simulink model "PX4ExtMsgSender"  (R2020b)
settings: Solver=ode4  StartTime=0.0  StopTime=inf  FixedStep=0.005  RelTol=1e-3
PreLoadFcn:
  | filepath  = fileparts(get_param(bdroot, 'FileName'))
  | cd(filepath);
undefined symbols (not defined in the file or in its folder): Busy, Earth, Wait, WGS84
libraries: etargetslib x6, slrealtimeiplib x3, dspnetwork x2, aerolibanimutils x1, aerolibtransform2 x1
settings Model: SimulationMode=accelerator  Creator=dream  LastModifiedBy=dzl20201126
settings DataIOCC: ReturnWorkspaceOutputs=off
settings DebuggingCC: ArithmeticOperatorsInVariantConditions=warning
settings SFSimCC: SimUseLocalCustomCode=off  CustomCodeUndefinedFunction=UseInterfaceOnly
settings RTWCC: RTWUseLocalCustomCode=off

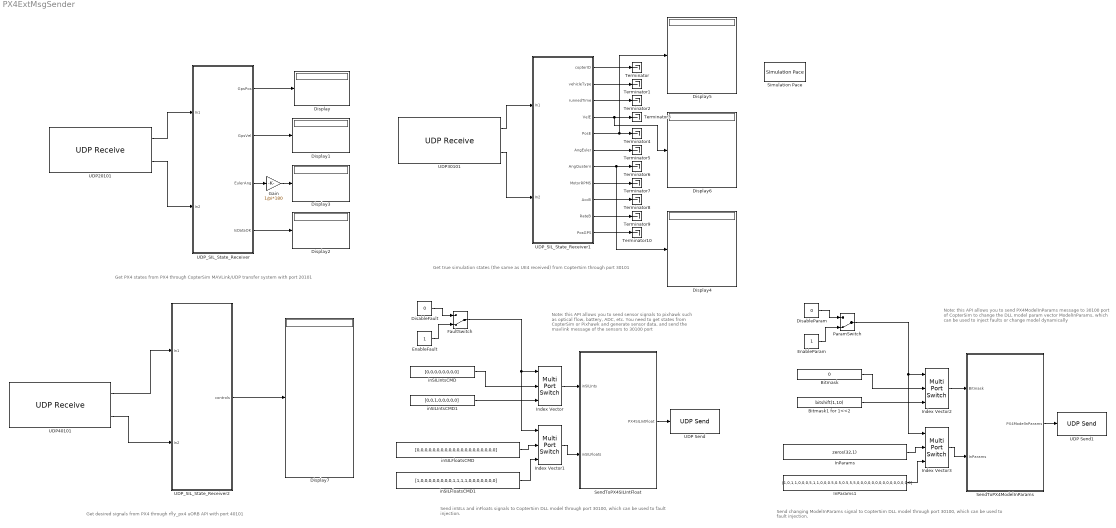
== system PX4ExtMsgSender ==
  note: Get PX4 states from PX4 through CopterSim MAVLink/UDP transfer system with port 20101
  note: Get true simulation states (the same as UE4 received) from CopterSim through port 30101
  note: Get desired signals from PX4 through rfly_px4 uORB API with port 40101
  note: Send inSILs and inFloats signals to CopterSim DLL model through port 30100, which can be used to fault injection.
  note: Note: this API allows you to send sensor signals to pixhawk such as optical flow, battery, ADC, etc. You need to get states from CopterSim or Pixhawk and generate sensor data, and send the mavlink message of the sensors to 30100 port
  note: Note: this API allows you to send PX4ModelInParams message to 30100 port of CopterSim to change the DLL model param vector ModelInParams, which can be used to inject faults or change model dynamically
  note: Send changing ModelInParams signal to CopterSim DLL model through port 30100, which can be used to fault injection.
  Bitmask : Constant  Value=0  OutDataTypeStr=int32
  Bitmask1 for 1<<2 : Constant  Value=bitshift(1,10)  OutDataTypeStr=int32
  DisableFault : Constant  Value=0
  DisableParam : Constant  Value=0
  Display{,1..7} (8 alike) : Display
  EnableFault : Constant
  EnableParam : Constant
  FaultSwitch : ManualSwitch  CurrentSetting=0
  Gain : Gain  Gain=1/pi*180
  InParams : Constant  Value=zeros(32,1)  OutDataTypeStr=single
  InParams1 : Constant  Value=[1,0,1,1,0,0,0,5,1,1,0,0,0.5,0.5,0.5,5,5,0,0,0,0,0,0,0,0,0,0,0,0,0,0,0]  OutDataTypeStr=single
  Index Vector{,1..3} (4 alike) : MultiPortSwitch  DataPortOrder=Zero-based contiguous  Inputs=2  zeroidx=on
  ParamSwitch : ManualSwitch  CurrentSetting=0
  SendToPX4ModelInParams : Subsystem
  SendToPX4SILIntFloat : Subsystem
  Simulation Pace : aerolibanimutils/Simulation Pace  SimulationPace=1  SleepMode=Busy-Wait  OutputPaceError=off  SampleTime=-1
  Terminator{,1..10} (11 alike) : Terminator
  UDP Send : dspnetwork/UDP Send  remoteURL='127.0.0.1'  remotePort=30100  localURL='0.0.0.0'  localPortSource=Automatically determine  localPort=-1  sendBufferSize=8192  sampletime=-1  blockPlatform=[]  separateLengthPort=0
  UDP Send1 : dspnetwork/UDP Send  remoteURL='127.0.0.1'  remotePort=30100  localURL='0.0.0.0'  localPortSource=Automatically determine  localPort=-1  sendBufferSize=8192  sampletime=-1  blockPlatform=[]  separateLengthPort=0
  UDP20101 : slrealtimeiplib/UDP Receive  useHostTargetConn=on  ipAddress=10.10.10.15  localPort=20101  rcvWidth=125  rcvFmAny=on  fmAddress=0.0.0.0  rcvMulticast=off  multicastAddress={}  sampleTime=-1
      settings: SourceProductBaseCode=XP
  UDP30101 : slrealtimeiplib/UDP Receive  useHostTargetConn=on  ipAddress=10.10.10.15  localPort=30101  rcvWidth=250  rcvFmAny=on  fmAddress=0.0.0.0  rcvMulticast=off  multicastAddress={}  sampleTime=-1
      settings: SourceProductBaseCode=XP
  UDP40101 : slrealtimeiplib/UDP Receive  useHostTargetConn=on  ipAddress=10.10.10.15  localPort=40101  rcvWidth=120  rcvFmAny=on  fmAddress=0.0.0.0  rcvMulticast=off  multicastAddress={}  sampleTime=-1
      settings: SourceProductBaseCode=XP
  UDP_SIL_State_Receiver : Subsystem
  UDP_SIL_State_Receiver1 : Subsystem
  UDP_SIL_State_Receiver2 : Subsystem
  inSILFloatsCMD : Constant  Value=[0,0,0,0,0,0,0,0,0,0,0,0,0,0,0,0,0,0,0,0]  OutDataTypeStr=single
  inSILFloatsCMD1 : Constant  Value=[1,0,0,0,0,0,0,0,0,1,1,1,1,0,0,0,0,0,0,0]  OutDataTypeStr=single
  inSILIntsCMD : Constant  Value=[0,0,0,0,0,0,0,0]  OutDataTypeStr=int32
  inSILIntsCMD1 : Constant  Value=[0,0,1,0,0,0,0,0]  OutDataTypeStr=int32
  wires:
  UDP20101/1 -> UDP_SIL_State_Receiver/1(In1)
  UDP20101/2 -> UDP_SIL_State_Receiver/2(In2)
  UDP_SIL_State_Receiver/1(GpsPos) -> Display/1
  UDP_SIL_State_Receiver/2(GpsVel) -> Display1/1
  UDP_SIL_State_Receiver/3(EulerAng) -> Gain/1
  Gain/1 -> Display3/1
  UDP_SIL_State_Receiver/4(IsDataOK) -> Display2/1
  UDP_SIL_State_Receiver1/8(MotorRPMS) -> Terminator7/1
  UDP_SIL_State_Receiver1/2(vehicleType) -> Terminator1/1
  UDP_SIL_State_Receiver1/9(AccB) -> Terminator8/1
  UDP_SIL_State_Receiver1/11(PosGPS) -> Terminator10/1
  UDP30101/2 -> UDP_SIL_State_Receiver1/2(In2)
  UDP_SIL_State_Receiver1/5(PosE) -> Display5/1, Terminator4/1
  UDP_SIL_State_Receiver1/6(AngEuler) -> Terminator5/1
  UDP_SIL_State_Receiver1/7(AngQuatern) -> Display4/1, Terminator6/1
  UDP_SIL_State_Receiver1/4(VelE) -> Display6/1, Terminator3/1
  SendToPX4SILIntFloat/1(PX4SILIntFloat) -> UDP Send/1
  UDP_SIL_State_Receiver1/3(runnedTime) -> Terminator2/1
  UDP_SIL_State_Receiver1/1(copterID) -> Terminator/1
  Index Vector1/1 -> SendToPX4SILIntFloat/2(inSILFloats)
  UDP30101/1 -> UDP_SIL_State_Receiver1/1(In1)
  DisableFault/1 -> FaultSwitch/1
  inSILFloatsCMD/1 -> Index Vector1/2
  inSILFloatsCMD1/1 -> Index Vector1/3
  Index Vector/1 -> SendToPX4SILIntFloat/1(inSILInts)
  inSILIntsCMD/1 -> Index Vector/2
  UDP_SIL_State_Receiver1/10(RateB) -> Terminator9/1
  EnableFault/1 -> FaultSwitch/2
  FaultSwitch/1 -> Index Vector1/1, Index Vector/1
  inSILIntsCMD1/1 -> Index Vector/3
  UDP40101/1 -> UDP_SIL_State_Receiver2/1(In1)
  UDP40101/2 -> UDP_SIL_State_Receiver2/2(In2)
  UDP_SIL_State_Receiver2/1(controls) -> Display7/1
  Index Vector2/1 -> SendToPX4ModelInParams/1(Bitmask)
  Bitmask1 for 1<<2/1 -> Index Vector2/3
  InParams/1 -> Index Vector3/2
  EnableParam/1 -> ParamSwitch/2
  InParams1/1 -> Index Vector3/3
  Bitmask/1 -> Index Vector2/2
  DisableParam/1 -> ParamSwitch/1
  ParamSwitch/1 -> Index Vector3/1, Index Vector2/1
  SendToPX4ModelInParams/1(PX4ModelInParams) -> UDP Send1/1
  Index Vector3/1 -> SendToPX4ModelInParams/2(InParams)

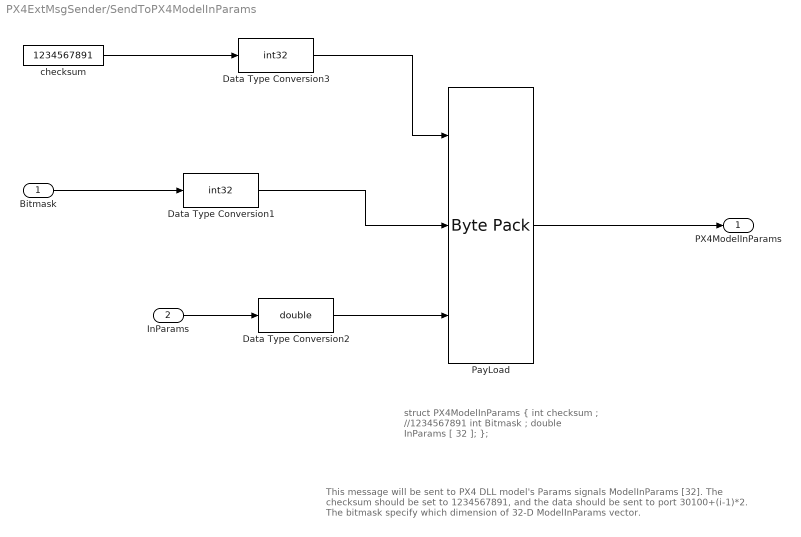
== system PX4ExtMsgSender/SendToPX4ModelInParams ==
  note: struct PX4ModelInParams {
      | int checksum ; //1234567891
      | int Bitmask ;
      | double InParams [ 32 ];
      | };
  note: This message will be sent to PX4 DLL model's Params signals ModelInParams [32].
      | The checksum should be set to 1234567891, and the data should be sent to port 30100+(i-1)*2.
      | The bitmask specify which dimension of 32-D ModelInParams vector.
  Bitmask : Inport  OutDataTypeStr=int32  PortDimensions=1
  InParams : Inport  Port=2  OutDataTypeStr=single  PortDimensions=32
  Data Type Conversion1 : DataTypeConversion  OutDataTypeStr=int32
  Data Type Conversion2 : DataTypeConversion  OutDataTypeStr=double
  Data Type Conversion3 : DataTypeConversion  OutDataTypeStr=int32
  PayLoad : etargetslib/Byte Pack  datatypes={'int32','int32','double'}  byteAlign=4
  checksum : Constant  Value=1234567891  OutDataTypeStr=Inherit: Inherit via back propagation
  PX4ModelInParams : Outport  OutDataTypeStr=uint8  VectorParamsAs1DForOutWhenUnconnected=off
  wires:
  InParams/1 -> Data Type Conversion2/1
  Bitmask/1 -> Data Type Conversion1/1
  PayLoad/1 -> PX4ModelInParams/1
  Data Type Conversion1/1 -> PayLoad/2
  Data Type Conversion2/1 -> PayLoad/3
  checksum/1 -> Data Type Conversion3/1
  Data Type Conversion3/1 -> PayLoad/1

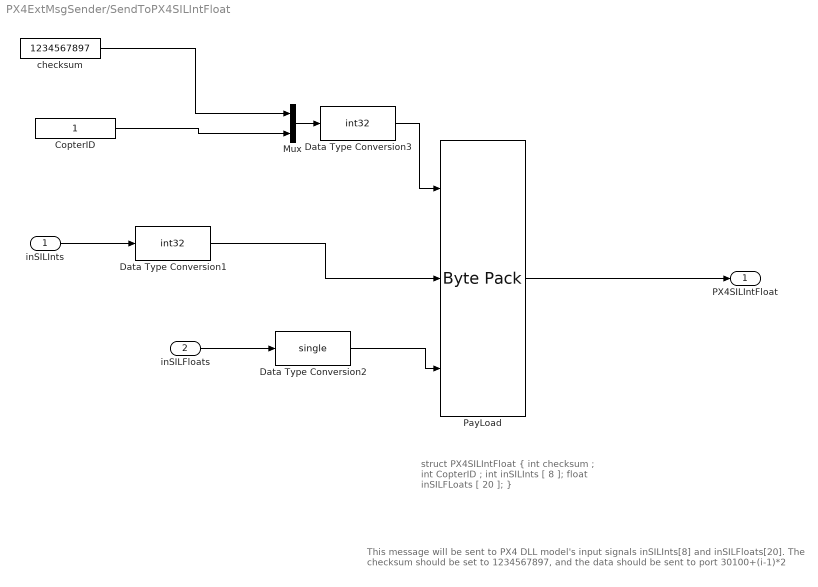
== system PX4ExtMsgSender/SendToPX4SILIntFloat ==
  note: struct PX4SILIntFloat {
      | int checksum ;
      | int CopterID ;
      | int inSILInts [ 8 ];
      | float inSILFLoats [ 20 ];
      | }
  note: This message will be sent to PX4 DLL model's input signals inSILInts[8] and inSILFloats[20].
      | The checksum should be set to 1234567897, and the data should be sent to port 30100+(i-1)*2
  inSILInts : Inport  OutDataTypeStr=int32  PortDimensions=8
  inSILFloats : Inport  Port=2  OutDataTypeStr=single  PortDimensions=20
  CopterID : Constant  OutDataTypeStr=Inherit: Inherit via back propagation
  Data Type Conversion1 : DataTypeConversion  OutDataTypeStr=int32
  Data Type Conversion2 : DataTypeConversion  OutDataTypeStr=single
  Data Type Conversion3 : DataTypeConversion  OutDataTypeStr=int32
  Mux : Mux  Inputs=2
  PayLoad : etargetslib/Byte Pack  datatypes={'int32','int32','single'}  byteAlign=8
  checksum : Constant  Value=1234567897  OutDataTypeStr=Inherit: Inherit via back propagation
  PX4SILIntFloat : Outport  OutDataTypeStr=uint8  PortDimensions=120  VectorParamsAs1DForOutWhenUnconnected=off
  wires:
  inSILFloats/1 -> Data Type Conversion2/1
  inSILInts/1 -> Data Type Conversion1/1
  PayLoad/1 -> PX4SILIntFloat/1
  Data Type Conversion1/1 -> PayLoad/2
  Data Type Conversion2/1 -> PayLoad/3
  checksum/1 -> Mux/1
  Mux/1 -> Data Type Conversion3/1
  Data Type Conversion3/1 -> PayLoad/1
  CopterID/1 -> Mux/2

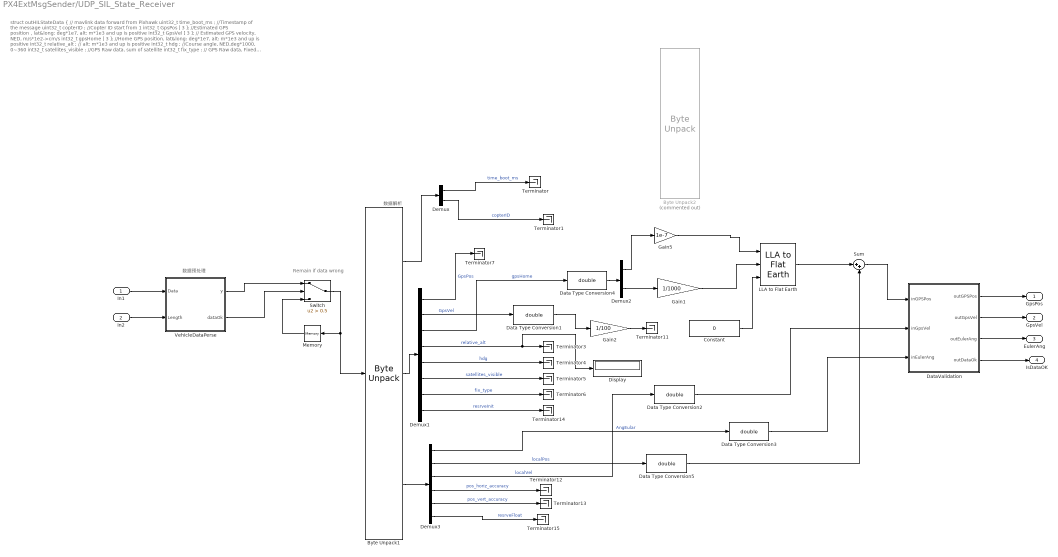
== system PX4ExtMsgSender/UDP_SIL_State_Receiver ==
  note: 数据解析
  note: 数据预处理
  note: Remain if data wrong
  note: struct outHILStateData { // mavlink data forward from Pixhawk
      | uint32_t time_boot_ms ; //Timestamp of the message
      | uint32_t copterID ; //Copter ID start from 1
      | int32_t GpsPos [ 3 ]; //Estimated GPS position，lat&long: deg*1e7, alt: m*1e3 and up is positive
      | int32_t GpsVel [ 3 ]; // Estimated GPS velocity, NED, m/s*1e2->cm/s
      | int32_t gpsHome [ 3 ]; //Home GPS position, lat&long: deg*1e7, alt: m*1e3 and up is positive
      | int32_t relative_alt ; // alt: m*1e3 and up is positive
      | int32_t hdg ; //Course angle, NED,deg*1000, 0~360
      | int32_t satellites_visible ; //GPS Raw data, sum of satellite
      | int32_t fix_type ; // GPS Raw data, Fixed type, 3 for fixed (good precision)
      | int32_t resrveInit ; //Int, reserve for the future use
      | float AngEular [ 3 ]; //Estimated Euler angle, unit: rad/s
      | float localPos [ 3 ]; //Estimated locoal position, NED, unit: m
      | float localVel [ 3 ]; // Estimated locoal velocity, NED, unit: m/s
      | float pos_horiz_accuracy ; // GPS horizontal accuracy, unit: m
      | float pos_vert_accuracy ; // GPS vertical accuracy, unit: m
      | float resrveFloat ; //float, reserve for the future use
      | }
  In1 : Inport
  In2 : Inport  Port=2
  Byte Unpack1 : etargetslib/Byte Unpack  dimensions={2,14,12}  datatypes={'uint32','int32','single'}  byteAlign=8
  Byte Unpack2 : etargetslib/Byte Unpack  Commented=on  dimensions={1,1,1,3,3,3,4,8,3,3,3}  datatypes={'int32','int32','double','single','single','single','single','single','single','single','double'}  byteAlign=1
  Constant : Constant  Value=0
  Data Type Conversion{1..5} (5 alike) : DataTypeConversion  OutDataTypeStr=double
  DataValidation : MATLAB Function  TreatAsAtomicUnit=on
  Demux : Demux  Outputs=2
  Demux1 : Demux  Outputs=[3,3,3,1,1,1,1,1]
  Demux2 : Demux  Outputs=[2,1]
  Demux3 : Demux  Outputs=[3,3,3,1,1,1]
  Display : Display
  Gain1 : Gain  Gain=1/1000
  Gain2 : Gain  Gain=1/100
  Gain5 : Gain  Gain=1e-7
  LLA to Flat Earth : aerolibtransform2/LLA to Flat Earth  units=Metric (MKS)  ptype=Earth (WGS84)  F=1/298.257223563  R=6378137  refPosPort=off  LL0=[40.1540302 116.259368300000]  psi=0
      settings: SourceProductBaseCode=AE
  Memory : Memory  InitialCondition=uint8(zeros(112,1))
  Sum : Sum  Inputs=|++
  Switch : Switch  Criteria=u2 > Threshold  Threshold=0.5
  Terminator{,1,3..7,11..15} (12 alike) : Terminator
  VehicleDataPerse : MATLAB Function  TreatAsAtomicUnit=on
  GpsPos : Outport  VectorParamsAs1DForOutWhenUnconnected=off
  GpsVel : Outport  Port=2  VectorParamsAs1DForOutWhenUnconnected=off
  EulerAng : Outport  Port=3  VectorParamsAs1DForOutWhenUnconnected=off
  IsDataOK : Outport  Port=4  VectorParamsAs1DForOutWhenUnconnected=off
  wires:
  VehicleDataPerse/2(dataOk) -> Switch/2
  In2/1 -> VehicleDataPerse/2(Length)
  In1/1 -> VehicleDataPerse/1(Data)
  VehicleDataPerse/1(y) -> Switch/1
  Switch/1 -> Memory/1, Byte Unpack1/1
  Memory/1 -> Switch/3
  Byte Unpack1/1 -> Demux/1
  Demux/1 -> Terminator/1  "time_boot_ms"
  Demux/2 -> Terminator1/1  "copterID"
  Byte Unpack1/2 -> Demux1/1
  Demux1/2 -> Data Type Conversion1/1  "GpsVel"
  Demux2/1 -> Gain5/1
  Demux2/2 -> Gain1/1
  Gain1/1 -> LLA to Flat Earth/2
  Demux1/1 -> Terminator7/1  "GpsPos"
  LLA to Flat Earth/1 -> Sum/1
  Data Type Conversion1/1 -> Gain2/1
  Data Type Conversion3/1 -> DataValidation/3(inEulerAng)
  Gain5/1 -> LLA to Flat Earth/1
  Data Type Conversion4/1 -> Demux2/1
  Byte Unpack1/3 -> Demux3/1
  Demux1/3 -> Data Type Conversion4/1  "gpsHome"
  Demux1/4 -> Display/1, Terminator3/1  "relative_alt"
  Demux1/5 -> Terminator4/1  "hdg"
  Demux1/6 -> Terminator5/1  "satellites_visible"
  Demux1/7 -> Terminator6/1  "fix_type"
  Demux3/1 -> Data Type Conversion3/1  "AngEular"
  Demux3/2 -> Data Type Conversion5/1  "localPos"
  Demux3/3 -> Data Type Conversion2/1  "localVel"
  Demux3/4 -> Terminator12/1  "pos_horiz_accuracy"
  Demux3/5 -> Terminator13/1  "pos_vert_accuracy"
  Demux1/8 -> Terminator14/1  "resrveInit"
  Demux3/6 -> Terminator15/1  "resrveFloat"
  Constant/1 -> LLA to Flat Earth/3
  DataValidation/1(outGPSPos) -> GpsPos/1
  DataValidation/2(outGpsVel) -> GpsVel/1
  DataValidation/3(outEulerAng) -> EulerAng/1
  DataValidation/4(outDataOk) -> IsDataOK/1
  Data Type Conversion2/1 -> DataValidation/2(inGpsVel)
  Gain2/1 -> Terminator11/1
  Data Type Conversion5/1 -> Sum/2
  Sum/1 -> DataValidation/1(inGPSPos)

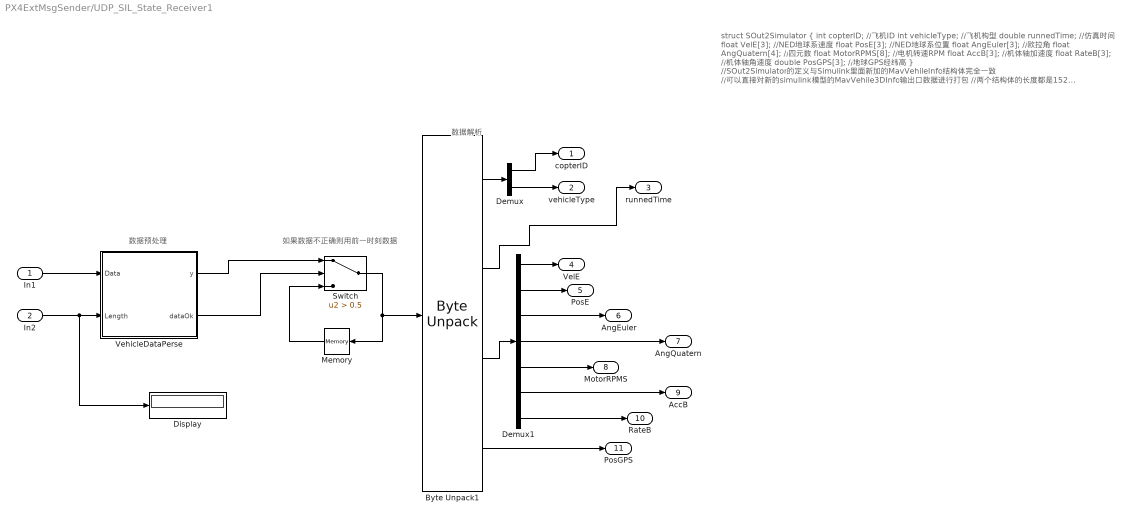
== system PX4ExtMsgSender/UDP_SIL_State_Receiver1 ==
  note: 数据解析
  note: 数据预处理
  note: 如果数据不正确则用前一时刻数据
  note: struct SOut2Simulator
      | {
      | int copterID; //飞机ID
      | int vehicleType; //飞机构型
      | double runnedTime; //仿真时间
      | float VelE[3]; //NED地球系速度
      | float PosE[3]; //NED地球系位置
      | float AngEuler[3]; //欧拉角
      | float AngQuatern[4]; //四元数
      | float MotorRPMS[8]; //电机转速RPM
      | float AccB[3]; //机体轴加速度
      | float RateB[3]; //机体轴角速度
      | double PosGPS[3]; //地球GPS经纬高
      | }
      |
      | //SOut2Simulator的定义与Simulink里面新加的MavVehileInfo结构体完全一致
      | //可以直接对新的simulink模型的MavVehile3DInfo输出口数据进行打包
      | //两个结构体的长度都是152
      | sizeof(SOut2Simulator) = sizeof(MavVehileInfo) = 152
      |
      | 打包封装的结构体为
      | typedef struct _netDataShort
      | {
      | TargetType tg; //这里目前随便填，写1即可 uint32
      | int len; //这个长度为传输结构体长度，目前是152
      | char payload[192]; //这里面前152位存放了SOut2Simulator结构体数据，后面的40位保留
      | }netDataShort;
      |
      | //UDP包的总长度为200
      | sizeof(netDataShort) = 200
      |
      | //发送的UDP端口号为：20010
  In1 : Inport
  In2 : Inport  Port=2
  Byte Unpack1 : etargetslib/Byte Unpack  dimensions={2,1,27,3}  datatypes={'int32','double','single','double'}  byteAlign=8
  Demux : Demux  Outputs=2
  Demux1 : Demux  Outputs=[3,3,3,4,8,3,3]
  Display : Display
  Memory : Memory  InitialCondition=uint8(zeros(152,1))
  Switch : Switch  Criteria=u2 > Threshold  Threshold=0.5
  VehicleDataPerse : MATLAB Function  TreatAsAtomicUnit=on
  copterID : Outport  VectorParamsAs1DForOutWhenUnconnected=off
  vehicleType : Outport  Port=2  VectorParamsAs1DForOutWhenUnconnected=off
  runnedTime : Outport  Port=3  VectorParamsAs1DForOutWhenUnconnected=off
  VelE : Outport  Port=4  VectorParamsAs1DForOutWhenUnconnected=off
  PosE : Outport  Port=5  VectorParamsAs1DForOutWhenUnconnected=off
  AngEuler : Outport  Port=6  VectorParamsAs1DForOutWhenUnconnected=off
  AngQuatern : Outport  Port=7  VectorParamsAs1DForOutWhenUnconnected=off
  MotorRPMS : Outport  Port=8  VectorParamsAs1DForOutWhenUnconnected=off
  AccB : Outport  Port=9  VectorParamsAs1DForOutWhenUnconnected=off
  RateB : Outport  Port=10  VectorParamsAs1DForOutWhenUnconnected=off
  PosGPS : Outport  Port=11  VectorParamsAs1DForOutWhenUnconnected=off
  wires:
  VehicleDataPerse/2(dataOk) -> Switch/2
  In2/1 -> Display/1, VehicleDataPerse/2(Length)
  In1/1 -> VehicleDataPerse/1(Data)
  VehicleDataPerse/1(y) -> Switch/1
  Switch/1 -> Memory/1, Byte Unpack1/1
  Memory/1 -> Switch/3
  Byte Unpack1/1 -> Demux/1
  Demux/1 -> copterID/1
  Demux/2 -> vehicleType/1
  Byte Unpack1/2 -> runnedTime/1
  Byte Unpack1/3 -> Demux1/1
  Demux1/1 -> VelE/1
  Demux1/2 -> PosE/1
  Demux1/3 -> AngEuler/1
  Demux1/4 -> AngQuatern/1
  Demux1/5 -> MotorRPMS/1
  Demux1/6 -> AccB/1
  Demux1/7 -> RateB/1
  Byte Unpack1/4 -> PosGPS/1

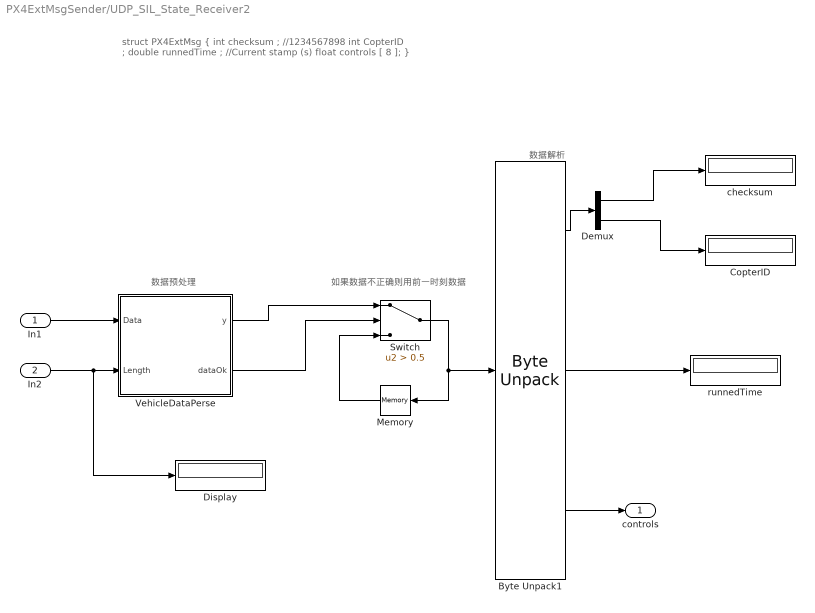
== system PX4ExtMsgSender/UDP_SIL_State_Receiver2 ==
  note: struct PX4ExtMsg {
      | int checksum ; //1234567898
      | int CopterID ;
      | double runnedTime ; //Current stamp (s)
      | float controls [ 8 ];
      | }
  note: 数据解析
  note: 数据预处理
  note: 如果数据不正确则用前一时刻数据
  In1 : Inport
  In2 : Inport  Port=2
  Byte Unpack1 : etargetslib/Byte Unpack  dimensions={2,1,8}  datatypes={'int32','double','single'}  byteAlign=8
  CopterID : Display
  Demux : Demux  Outputs=2
  Display : Display
  Memory : Memory  InitialCondition=uint8(zeros(48,1))
  Switch : Switch  Criteria=u2 > Threshold  Threshold=0.5
  VehicleDataPerse : MATLAB Function  TreatAsAtomicUnit=on
  checksum : Display
  runnedTime : Display
  controls : Outport  VectorParamsAs1DForOutWhenUnconnected=off
  wires:
  VehicleDataPerse/2(dataOk) -> Switch/2
  In2/1 -> Display/1, VehicleDataPerse/2(Length)
  In1/1 -> VehicleDataPerse/1(Data)
  VehicleDataPerse/1(y) -> Switch/1
  Switch/1 -> Memory/1, Byte Unpack1/1
  Memory/1 -> Switch/3
  Byte Unpack1/1 -> Demux/1
  Demux/1 -> checksum/1
  Demux/2 -> CopterID/1
  Byte Unpack1/2 -> runnedTime/1
  Byte Unpack1/3 -> controls/1

== matlab function PX4ExtMsgSender/UDP_SIL_State_Receiver1/VehicleDataPerse ==
  data: Data input; y output uint8 size=[152,1]; Length input; dataOk output
function [y,dataOk] = fcn(Data,Length)
y=uint8(zeros(152,1));
dataOk = 0;
if Length ~= 200
    return;
end
len = typecast(Data(5:8), 'int32');

if len ~= 152
   return; 
end

y = Data(9:160);
dataOk = 1;

== matlab function PX4ExtMsgSender/UDP_SIL_State_Receiver/DataValidation ==
  data: inGPSPos input; outGPSPos output; inGpsVel input; inEulerAng input; outGpsVel output; outEulerAng output; outDataOk output
function [outGPSPos,outGpsVel,outEulerAng,outDataOk] = fcn(inGPSPos,inGpsVel,inEulerAng)

outGPSPos = [0;0;0];
outGpsVel = [0;0;0];
outEulerAng = [0;0;0];
outDataOk = 0;

if(abs(inGPSPos(1))<10000)
    outGPSPos=inGPSPos;
    outGpsVel=inGpsVel;
    outEulerAng = inEulerAng;
    outDataOk = 1;
end

== matlab function PX4ExtMsgSender/UDP_SIL_State_Receiver2/VehicleDataPerse ==
  data: Data input; y output uint8 size=[48,1]; Length input; dataOk output
function [y,dataOk] = fcn(Data,Length)
y=uint8(zeros(48,1));
dataOk = 0;
if Length ~= 48
    return;
end
checksum=typecast(Data(1:4), 'int32');
if checksum ~= 1234567898
    return;
end

y = Data(1:48);
dataOk = 1;

== matlab function PX4ExtMsgSender/UDP_SIL_State_Receiver/VehicleDataPerse ==
  data: Data input; y output uint8; Length input; dataOk output
function [y,dataOk] = fcn(Data,Length)
y=uint8(zeros(112,1));
dataOk = 0;
if Length ~= 120
    return;
end
len = typecast(Data(5:8), 'int32');

if len ~= 112
   return; 
end

y = Data(9:120);
dataOk = 1;
